simulink model "qless_forgetting_factor_16x16"  (R2021a)
settings: Solver=FixedStepDiscrete  StartTime=0.0  StopTime=stoptime*inf  RelTol=1e-3
InitFcn:
  | qless_init_16chan_fi
undefined symbols (not defined in the file): fc, numArrayElements, physconst, srcAngles, sv, Ts
libraries: hdlsllib x137, commfilt2 x4, commrfcorlib x3, commsync2 x3, commrflib2 x2, commrandsrc3 x2, phasedtxrxlib x2, commdigbbndcpm2 x1, simulink x1, embreciprocals x1, commdigbbndpm3 x1
(part 2 of 22)

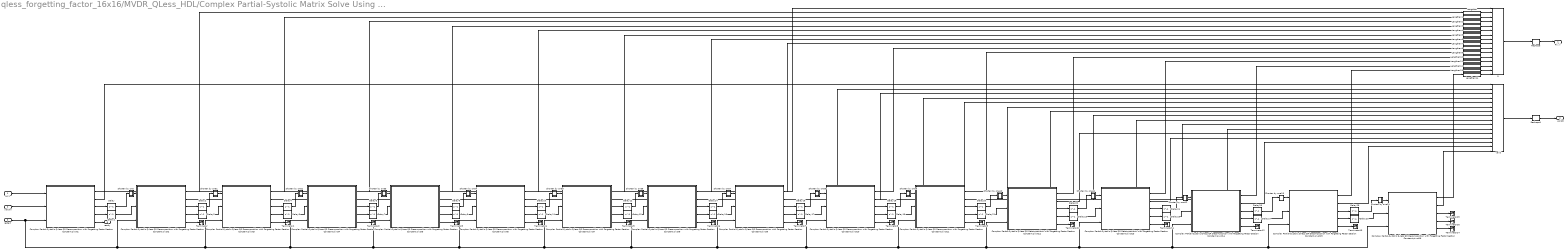
== system qless_forgetting_factor_16x16/MVDR_QLess_HDL/Complex Partial-Systolic Matrix Solve Using Q-less QR Decomposition with Forgetting Factor Manually Tiled n=16/Complex Partial-Systolic Q-less QR with Forgetting Factor/Complex Partial-Systolic Q-less QR with Forgetting Factor Manually tiled ==
  A(i,:) : Inport  PortDimensions=[1,n]
  validIn : Inport  Port=2  PortDimensions=1
  restart : Inport  Port=3  PortDimensions=1
  Complex Partial-Systolic Q-less QR Decomposition with Forgetting Factor Section Constant pivot1 : Subsystem  mask{n=n, forgettingFactor=forgettingFactor, pivot=1}
      mask prompts: n "fixed:emblib:ColumnsInA"; forgettingFactor "fixed:emblib:ForgettingFactor"
      mask DialogControl n Prompt: Number of columns in matrix A
      mask DialogControl forgettingFactor Prompt: Forgetting factor
  Complex Partial-Systolic Q-less QR Decomposition with Forgetting Factor Section Constant pivot10 : Subsystem  mask{n=n-9, forgettingFactor=forgettingFactor, pivot=1}
      mask prompts: n "fixed:emblib:ColumnsInA"; forgettingFactor "fixed:emblib:ForgettingFactor"
      mask DialogControl n Prompt: Number of columns in matrix A
      mask DialogControl forgettingFactor Prompt: Forgetting factor
  Complex Partial-Systolic Q-less QR Decomposition with Forgetting Factor Section Constant pivot11 : Subsystem  mask{n=n-10, forgettingFactor=forgettingFactor, pivot=1}
      mask prompts: n "fixed:emblib:ColumnsInA"; forgettingFactor "fixed:emblib:ForgettingFactor"
      mask DialogControl n Prompt: Number of columns in matrix A
      mask DialogControl forgettingFactor Prompt: Forgetting factor
  Complex Partial-Systolic Q-less QR Decomposition with Forgetting Factor Section Constant pivot12 : Subsystem  mask{n=n-11, forgettingFactor=forgettingFactor, pivot=1}
      mask prompts: n "fixed:emblib:ColumnsInA"; forgettingFactor "fixed:emblib:ForgettingFactor"
      mask DialogControl n Prompt: Number of columns in matrix A
      mask DialogControl forgettingFactor Prompt: Forgetting factor
  Complex Partial-Systolic Q-less QR Decomposition with Forgetting Factor Section Constant pivot13 : Subsystem  mask{n=n-12, forgettingFactor=forgettingFactor, pivot=1}
      mask prompts: n "fixed:emblib:ColumnsInA"; forgettingFactor "fixed:emblib:ForgettingFactor"
      mask DialogControl n Prompt: Number of columns in matrix A
      mask DialogControl forgettingFactor Prompt: Forgetting factor
  Complex Partial-Systolic Q-less QR Decomposition with Forgetting Factor Section Constant pivot14 : Subsystem  mask{n=n-13, forgettingFactor=forgettingFactor, pivot=1}
      mask prompts: n "fixed:emblib:ColumnsInA"; forgettingFactor "fixed:emblib:ForgettingFactor"
      mask DialogControl n Prompt: Number of columns in matrix A
      mask DialogControl forgettingFactor Prompt: Forgetting factor
  Complex Partial-Systolic Q-less QR Decomposition with Forgetting Factor Section Constant pivot15 : Subsystem  mask{n=n-14, forgettingFactor=forgettingFactor, pivot=1}
      mask prompts: n "fixed:emblib:ColumnsInA"; forgettingFactor "fixed:emblib:ForgettingFactor"
      mask DialogControl n Prompt: Number of columns in matrix A
      mask DialogControl forgettingFactor Prompt: Forgetting factor
  Complex Partial-Systolic Q-less QR Decomposition with Forgetting Factor Section Constant pivot16 : Subsystem  mask{n=n-15, forgettingFactor=forgettingFactor, pivot=1}
      mask prompts: n "fixed:emblib:ColumnsInA"; forgettingFactor "fixed:emblib:ForgettingFactor"
      mask DialogControl n Prompt: Number of columns in matrix A
      mask DialogControl forgettingFactor Prompt: Forgetting factor
  Complex Partial-Systolic Q-less QR Decomposition with Forgetting Factor Section Constant pivot2 : Subsystem  mask{n=n-1, forgettingFactor=forgettingFactor, pivot=1}
      mask prompts: n "fixed:emblib:ColumnsInA"; forgettingFactor "fixed:emblib:ForgettingFactor"
      mask DialogControl n Prompt: Number of columns in matrix A
      mask DialogControl forgettingFactor Prompt: Forgetting factor
  Complex Partial-Systolic Q-less QR Decomposition with Forgetting Factor Section Constant pivot3 : Subsystem  mask{n=n-2, forgettingFactor=forgettingFactor, pivot=1}
      mask prompts: n "fixed:emblib:ColumnsInA"; forgettingFactor "fixed:emblib:ForgettingFactor"
      mask DialogControl n Prompt: Number of columns in matrix A
      mask DialogControl forgettingFactor Prompt: Forgetting factor
  Complex Partial-Systolic Q-less QR Decomposition with Forgetting Factor Section Constant pivot4 : Subsystem  mask{n=n-3, forgettingFactor=forgettingFactor, pivot=1}
      mask prompts: n "fixed:emblib:ColumnsInA"; forgettingFactor "fixed:emblib:ForgettingFactor"
      mask DialogControl n Prompt: Number of columns in matrix A
      mask DialogControl forgettingFactor Prompt: Forgetting factor
  Complex Partial-Systolic Q-less QR Decomposition with Forgetting Factor Section Constant pivot5 : Subsystem  mask{n=n-4, forgettingFactor=forgettingFactor, pivot=1}
      mask prompts: n "fixed:emblib:ColumnsInA"; forgettingFactor "fixed:emblib:ForgettingFactor"
      mask DialogControl n Prompt: Number of columns in matrix A
      mask DialogControl forgettingFactor Prompt: Forgetting factor
  Complex Partial-Systolic Q-less QR Decomposition with Forgetting Factor Section Constant pivot6 : Subsystem  mask{n=n-5, forgettingFactor=forgettingFactor, pivot=1}
      mask prompts: n "fixed:emblib:ColumnsInA"; forgettingFactor "fixed:emblib:ForgettingFactor"
      mask DialogControl n Prompt: Number of columns in matrix A
      mask DialogControl forgettingFactor Prompt: Forgetting factor
  Complex Partial-Systolic Q-less QR Decomposition with Forgetting Factor Section Constant pivot7 : Subsystem  mask{n=n-6, forgettingFactor=forgettingFactor, pivot=1}
      mask prompts: n "fixed:emblib:ColumnsInA"; forgettingFactor "fixed:emblib:ForgettingFactor"
      mask DialogControl n Prompt: Number of columns in matrix A
      mask DialogControl forgettingFactor Prompt: Forgetting factor
  Complex Partial-Systolic Q-less QR Decomposition with Forgetting Factor Section Constant pivot8 : Subsystem  mask{n=n-7, forgettingFactor=forgettingFactor, pivot=1}
      mask prompts: n "fixed:emblib:ColumnsInA"; forgettingFactor "fixed:emblib:ForgettingFactor"
      mask DialogControl n Prompt: Number of columns in matrix A
      mask DialogControl forgettingFactor Prompt: Forgetting factor
  Complex Partial-Systolic Q-less QR Decomposition with Forgetting Factor Section Constant pivot9 : Subsystem  mask{n=n-8, forgettingFactor=forgettingFactor, pivot=1}
      mask prompts: n "fixed:emblib:ColumnsInA"; forgettingFactor "fixed:emblib:ForgettingFactor"
      mask DialogControl n Prompt: Number of columns in matrix A
      mask DialogControl forgettingFactor Prompt: Forgetting factor
  Delay{,1..29} (30 alike) : Delay  DelayLength=1
  Lengthen : Subsystem  mask{number_of_leading_zeros=1}
      mask prompts: number_of_leading_zeros "Number of leading zeros to add"
      mask Display: disp('Lengthen')
  Lengthen1 : Subsystem  mask{number_of_leading_zeros=2}
      mask prompts: number_of_leading_zeros "Number of leading zeros to add"
      mask Display: disp('Lengthen')
  Lengthen10 : Subsystem  mask{number_of_leading_zeros=11}
      mask prompts: number_of_leading_zeros "Number of leading zeros to add"
      mask Display: disp('Lengthen')
  Lengthen11 : Subsystem  mask{number_of_leading_zeros=12}
      mask prompts: number_of_leading_zeros "Number of leading zeros to add"
      mask Display: disp('Lengthen')
  Lengthen12 : Subsystem  mask{number_of_leading_zeros=13}
      mask prompts: number_of_leading_zeros "Number of leading zeros to add"
      mask Display: disp('Lengthen')
  Lengthen13 : Subsystem  mask{number_of_leading_zeros=14}
      mask prompts: number_of_leading_zeros "Number of leading zeros to add"
      mask Display: disp('Lengthen')
  Lengthen14 : Subsystem  mask{number_of_leading_zeros=15}
      mask prompts: number_of_leading_zeros "Number of leading zeros to add"
      mask Display: disp('Lengthen')
  Lengthen2 : Subsystem  mask{number_of_leading_zeros=3}
      mask prompts: number_of_leading_zeros "Number of leading zeros to add"
      mask Display: disp('Lengthen')
  Lengthen3 : Subsystem  mask{number_of_leading_zeros=4}
      mask prompts: number_of_leading_zeros "Number of leading zeros to add"
      mask Display: disp('Lengthen')
  Lengthen4 : Subsystem  mask{number_of_leading_zeros=5}
      mask prompts: number_of_leading_zeros "Number of leading zeros to add"
      mask Display: disp('Lengthen')
  Lengthen5 : Subsystem  mask{number_of_leading_zeros=6}
      mask prompts: number_of_leading_zeros "Number of leading zeros to add"
      mask Display: disp('Lengthen')
  Lengthen6 : Subsystem  mask{number_of_leading_zeros=7}
      mask prompts: number_of_leading_zeros "Number of leading zeros to add"
      mask Display: disp('Lengthen')
  Lengthen7 : Subsystem  mask{number_of_leading_zeros=8}
      mask prompts: number_of_leading_zeros "Number of leading zeros to add"
      mask Display: disp('Lengthen')
  Lengthen8 : Subsystem  mask{number_of_leading_zeros=9}
      mask prompts: number_of_leading_zeros "Number of leading zeros to add"
      mask Display: disp('Lengthen')
  Lengthen9 : Subsystem  mask{number_of_leading_zeros=10}
      mask prompts: number_of_leading_zeros "Number of leading zeros to add"
      mask Display: disp('Lengthen')
  R : Concatenate  NumInputs=16
  Reshape : Reshape  OutputDimensionality=Row vector (2-D)
  Reshape1 : Reshape  OutputDimensionality=Row vector (2-D)
  Shorten by one : MATLAB Function  TreatAsAtomicUnit=on
  Shorten by one1 : MATLAB Function  TreatAsAtomicUnit=on
  Shorten by one10 : MATLAB Function  TreatAsAtomicUnit=on
  Shorten by one11 : MATLAB Function  TreatAsAtomicUnit=on
  Shorten by one12 : MATLAB Function  TreatAsAtomicUnit=on
  Shorten by one13 : MATLAB Function  TreatAsAtomicUnit=on
  Shorten by one14 : MATLAB Function  TreatAsAtomicUnit=on
  Shorten by one2 : MATLAB Function  TreatAsAtomicUnit=on
  Shorten by one3 : MATLAB Function  TreatAsAtomicUnit=on
  Shorten by one4 : MATLAB Function  TreatAsAtomicUnit=on
  Shorten by one5 : MATLAB Function  TreatAsAtomicUnit=on
  Shorten by one6 : MATLAB Function  TreatAsAtomicUnit=on
  Shorten by one7 : MATLAB Function  TreatAsAtomicUnit=on
  Shorten by one8 : MATLAB Function  TreatAsAtomicUnit=on
  Shorten by one9 : MATLAB Function  TreatAsAtomicUnit=on
  Terminator{,1..16} (17 alike) : Terminator
  valid : Concatenate  NumInputs=16
  R(i,:).' : Outport  PortDimensions=[1,n*n]
  validR : Outport  Port=2  PortDimensions=[1,n]
  ready : Outport  Port=3  PortDimensions=1
  wires:
  Complex Partial-Systolic Q-less QR Decomposition with Forgetting Factor Section Constant pivot16/1("R(i, :)^T") -> Lengthen14/1(u)
  Lengthen14/1(y) -> R/16
  Shorten by one14/1(y) -> Complex Partial-Systolic Q-less QR Decomposition with Forgetting Factor Section Constant pivot16/1("A(i, :)^T")
  Delay28/1 -> Shorten by one14/1(u)
  Shorten by one13/1(y) -> Complex Partial-Systolic Q-less QR Decomposition with Forgetting Factor Section Constant pivot15/1("A(i, :)^T")
  Delay26/1 -> Shorten by one13/1(u)
  Shorten by one12/1(y) -> Complex Partial-Systolic Q-less QR Decomposition with Forgetting Factor Section Constant pivot14/1("A(i, :)^T")
  Delay24/1 -> Shorten by one12/1(u)
  Shorten by one11/1(y) -> Complex Partial-Systolic Q-less QR Decomposition with Forgetting Factor Section Constant pivot13/1("A(i, :)^T")
  Delay22/1 -> Shorten by one11/1(u)
  Shorten by one10/1(y) -> Complex Partial-Systolic Q-less QR Decomposition with Forgetting Factor Section Constant pivot12/1("A(i, :)^T")
  Delay20/1 -> Shorten by one10/1(u)
  Shorten by one9/1(y) -> Complex Partial-Systolic Q-less QR Decomposition with Forgetting Factor Section Constant pivot11/1("A(i, :)^T")
  Delay18/1 -> Shorten by one9/1(u)
  Shorten by one8/1(y) -> Complex Partial-Systolic Q-less QR Decomposition with Forgetting Factor Section Constant pivot10/1("A(i, :)^T")
  Delay16/1 -> Shorten by one8/1(u)
  Shorten by one7/1(y) -> Complex Partial-Systolic Q-less QR Decomposition with Forgetting Factor Section Constant pivot9/1("A(i, :)^T")
  Delay14/1 -> Shorten by one7/1(u)
  Shorten by one6/1(y) -> Complex Partial-Systolic Q-less QR Decomposition with Forgetting Factor Section Constant pivot8/1("A(i, :)^T")
  Delay12/1 -> Shorten by one6/1(u)
  Shorten by one5/1(y) -> Complex Partial-Systolic Q-less QR Decomposition with Forgetting Factor Section Constant pivot7/1("A(i, :)^T")
  Delay10/1 -> Shorten by one5/1(u)
  Shorten by one4/1(y) -> Complex Partial-Systolic Q-less QR Decomposition with Forgetting Factor Section Constant pivot6/1("A(i, :)^T")
  Delay8/1 -> Shorten by one4/1(u)
  Shorten by one3/1(y) -> Complex Partial-Systolic Q-less QR Decomposition with Forgetting Factor Section Constant pivot5/1("A(i, :)^T")
  Delay6/1 -> Shorten by one3/1(u)
  Delay4/1 -> Shorten by one2/1(u)
  Shorten by one2/1(y) -> Complex Partial-Systolic Q-less QR Decomposition with Forgetting Factor Section Constant pivot4/1("A(i, :)^T")
  Delay2/1 -> Shorten by one1/1(u)
  Shorten by one1/1(y) -> Complex Partial-Systolic Q-less QR Decomposition with Forgetting Factor Section Constant pivot3/1("A(i, :)^T")
  Shorten by one/1(y) -> Complex Partial-Systolic Q-less QR Decomposition with Forgetting Factor Section Constant pivot2/1("A(i, :)^T")
  Lengthen13/1(y) -> R/15
  Lengthen12/1(y) -> R/14
  Lengthen11/1(y) -> R/13
  Lengthen10/1(y) -> R/12
  Lengthen9/1(y) -> R/11
  Lengthen8/1(y) -> R/10
  Lengthen7/1(y) -> R/9
  Lengthen6/1(y) -> R/8
  Lengthen5/1(y) -> R/7
  Lengthen4/1(y) -> R/6
  Lengthen3/1(y) -> R/5
  Lengthen2/1(y) -> R/4
  Lengthen1/1(y) -> R/3
  Lengthen/1(y) -> R/2
  Reshape1/1 -> validR/1
  restart/1 -> Complex Partial-Systolic Q-less QR Decomposition with Forgetting Factor Section Constant pivot1/3(restart), Complex Partial-Systolic Q-less QR Decomposition with Forgetting Factor Section Constant pivot16/3(restart), Complex Partial-Systolic Q-less QR Decomposition with Forgetting Factor Section Constant pivot15/3(restart), Complex Partial-Systolic Q-less QR Decomposition with Forgetting Factor Section Constant pivot14/3(restart), Complex Partial-Systolic Q-less QR Decomposition with Forgetting Factor Section Constant pivot13/3(restart), Complex Partial-Systolic Q-less QR Decomposition with Forgetting Factor Section Constant pivot12/3(restart), Complex Partial-Systolic Q-less QR Decomposition with Forgetting Factor Section Constant pivot11/3(restart), Complex Partial-Systolic Q-less QR Decomposition with Forgetting Factor Section Constant pivot10/3(restart), Complex Partial-Systolic Q-less QR Decomposition with Forgetting Factor Section Constant pivot9/3(restart), Complex Partial-Systolic Q-less QR Decomposition with Forgetting Factor Section Constant pivot8/3(restart), Complex Partial-Systolic Q-less QR Decomposition with Forgetting Factor Section Constant pivot7/3(restart), Complex Partial-Systolic Q-less QR Decomposition with Forgetting Factor Section Constant pivot6/3(restart), Complex Partial-Systolic Q-less QR Decomposition with Forgetting Factor Section Constant pivot5/3(restart), Complex Partial-Systolic Q-less QR Decomposition with Forgetting Factor Section Constant pivot4/3(restart), Complex Partial-Systolic Q-less QR Decomposition with Forgetting Factor Section Constant pivot3/3(restart), Complex Partial-Systolic Q-less QR Decomposition with Forgetting Factor Section Constant pivot2/3(restart)
  valid/1 -> Reshape1/1
  Reshape/1 -> R(i,:).'/1
  R/1 -> Reshape/1
  Complex Partial-Systolic Q-less QR Decomposition with Forgetting Factor Section Constant pivot16/2(validR) -> valid/16
  Complex Partial-Systolic Q-less QR Decomposition with Forgetting Factor Section Constant pivot15/2(validR) -> valid/15
  Complex Partial-Systolic Q-less QR Decomposition with Forgetting Factor Section Constant pivot15/1("R(i, :)^T") -> Lengthen13/1(u)
  Complex Partial-Systolic Q-less QR Decomposition with Forgetting Factor Section Constant pivot14/2(validR) -> valid/14
  Complex Partial-Systolic Q-less QR Decomposition with Forgetting Factor Section Constant pivot14/1("R(i, :)^T") -> Lengthen12/1(u)
  Complex Partial-Systolic Q-less QR Decomposition with Forgetting Factor Section Constant pivot13/2(validR) -> valid/13
  Complex Partial-Systolic Q-less QR Decomposition with Forgetting Factor Section Constant pivot13/1("R(i, :)^T") -> Lengthen11/1(u)
  Complex Partial-Systolic Q-less QR Decomposition with Forgetting Factor Section Constant pivot12/2(validR) -> valid/12
  Complex Partial-Systolic Q-less QR Decomposition with Forgetting Factor Section Constant pivot12/1("R(i, :)^T") -> Lengthen10/1(u)
  Delay29/1 -> Complex Partial-Systolic Q-less QR Decomposition with Forgetting Factor Section Constant pivot16/2(validIn)
  Delay27/1 -> Complex Partial-Systolic Q-less QR Decomposition with Forgetting Factor Section Constant pivot15/2(validIn)
  Delay25/1 -> Complex Partial-Systolic Q-less QR Decomposition with Forgetting Factor Section Constant pivot14/2(validIn)
  Delay23/1 -> Complex Partial-Systolic Q-less QR Decomposition with Forgetting Factor Section Constant pivot13/2(validIn)
  Complex Partial-Systolic Q-less QR Decomposition with Forgetting Factor Section Constant pivot11/2(validR) -> valid/11
  Complex Partial-Systolic Q-less QR Decomposition with Forgetting Factor Section Constant pivot11/1("R(i, :)^T") -> Lengthen9/1(u)
  Complex Partial-Systolic Q-less QR Decomposition with Forgetting Factor Section Constant pivot10/2(validR) -> valid/10
  Complex Partial-Systolic Q-less QR Decomposition with Forgetting Factor Section Constant pivot10/1("R(i, :)^T") -> Lengthen8/1(u)
  Complex Partial-Systolic Q-less QR Decomposition with Forgetting Factor Section Constant pivot9/2(validR) -> valid/9
  Complex Partial-Systolic Q-less QR Decomposition with Forgetting Factor Section Constant pivot9/1("R(i, :)^T") -> Lengthen7/1(u)
  Complex Partial-Systolic Q-less QR Decomposition with Forgetting Factor Section Constant pivot8/2(validR) -> valid/8
  Complex Partial-Systolic Q-less QR Decomposition with Forgetting Factor Section Constant pivot8/1("R(i, :)^T") -> Lengthen6/1(u)
  Complex Partial-Systolic Q-less QR Decomposition with Forgetting Factor Section Constant pivot7/2(validR) -> valid/7
  Complex Partial-Systolic Q-less QR Decomposition with Forgetting Factor Section Constant pivot7/1("R(i, :)^T") -> Lengthen5/1(u)
  Delay21/1 -> Complex Partial-Systolic Q-less QR Decomposition with Forgetting Factor Section Constant pivot12/2(validIn)
  Delay19/1 -> Complex Partial-Systolic Q-less QR Decomposition with Forgetting Factor Section Constant pivot11/2(validIn)
  Delay17/1 -> Complex Partial-Systolic Q-less QR Decomposition with Forgetting Factor Section Constant pivot10/2(validIn)
  Delay15/1 -> Complex Partial-Systolic Q-less QR Decomposition with Forgetting Factor Section Constant pivot9/2(validIn)
  Complex Partial-Systolic Q-less QR Decomposition with Forgetting Factor Section Constant pivot6/2(validR) -> valid/6
  Complex Partial-Systolic Q-less QR Decomposition with Forgetting Factor Section Constant pivot6/1("R(i, :)^T") -> Lengthen4/1(u)
  Delay13/1 -> Complex Partial-Systolic Q-less QR Decomposition with Forgetting Factor Section Constant pivot8/2(validIn)
  Delay11/1 -> Complex Partial-Systolic Q-less QR Decomposition with Forgetting Factor Section Constant pivot7/2(validIn)
  Delay9/1 -> Complex Partial-Systolic Q-less QR Decomposition with Forgetting Factor Section Constant pivot6/2(validIn)
  Complex Partial-Systolic Q-less QR Decomposition with Forgetting Factor Section Constant pivot5/2(validR) -> valid/5
  Complex Partial-Systolic Q-less QR Decomposition with Forgetting Factor Section Constant pivot5/1("R(i, :)^T") -> Lengthen3/1(u)
  Complex Partial-Systolic Q-less QR Decomposition with Forgetting Factor Section Constant pivot4/2(validR) -> valid/4
  Complex Partial-Systolic Q-less QR Decomposition with Forgetting Factor Section Constant pivot4/1("R(i, :)^T") -> Lengthen2/1(u)
  Complex Partial-Systolic Q-less QR Decomposition with Forgetting Factor Section Constant pivot3/2(validR) -> valid/3
  Complex Partial-Systolic Q-less QR Decomposition with Forgetting Factor Section Constant pivot3/1("R(i, :)^T") -> Lengthen1/1(u)
  Delay7/1 -> Complex Partial-Systolic Q-less QR Decomposition with Forgetting Factor Section Constant pivot5/2(validIn)
  Delay5/1 -> Complex Partial-Systolic Q-less QR Decomposition with Forgetting Factor Section Constant pivot4/2(validIn)
  Delay3/1 -> Complex Partial-Systolic Q-less QR Decomposition with Forgetting Factor Section Constant pivot3/2(validIn)
  Complex Partial-Systolic Q-less QR Decomposition with Forgetting Factor Section Constant pivot2/2(validR) -> valid/2
  Complex Partial-Systolic Q-less QR Decomposition with Forgetting Factor Section Constant pivot2/1("R(i, :)^T") -> Lengthen/1(u)
  Delay1/1 -> Complex Partial-Systolic Q-less QR Decomposition with Forgetting Factor Section Constant pivot2/2(validIn)
  Delay/1 -> Shorten by one/1(u)
  Complex Partial-Systolic Q-less QR Decomposition with Forgetting Factor Section Constant pivot1/2(validR) -> valid/1
  Complex Partial-Systolic Q-less QR Decomposition with Forgetting Factor Section Constant pivot1/1("R(i, :)^T") -> R/1
  Complex Partial-Systolic Q-less QR Decomposition with Forgetting Factor Section Constant pivot16/5(ready) -> Terminator14/1
  Complex Partial-Systolic Q-less QR Decomposition with Forgetting Factor Section Constant pivot15/5(ready) -> Terminator13/1
  Complex Partial-Systolic Q-less QR Decomposition with Forgetting Factor Section Constant pivot14/5(ready) -> Terminator12/1
  Complex Partial-Systolic Q-less QR Decomposition with Forgetting Factor Section Constant pivot13/5(ready) -> Terminator11/1
  Complex Partial-Systolic Q-less QR Decomposition with Forgetting Factor Section Constant pivot12/5(ready) -> Terminator10/1
  Complex Partial-Systolic Q-less QR Decomposition with Forgetting Factor Section Constant pivot11/5(ready) -> Terminator9/1
  Complex Partial-Systolic Q-less QR Decomposition with Forgetting Factor Section Constant pivot10/5(ready) -> Terminator8/1
  Complex Partial-Systolic Q-less QR Decomposition with Forgetting Factor Section Constant pivot9/5(ready) -> Terminator7/1
  Complex Partial-Systolic Q-less QR Decomposition with Forgetting Factor Section Constant pivot8/5(ready) -> Terminator6/1
  Complex Partial-Systolic Q-less QR Decomposition with Forgetting Factor Section Constant pivot7/5(ready) -> Terminator5/1
  Complex Partial-Systolic Q-less QR Decomposition with Forgetting Factor Section Constant pivot6/5(ready) -> Terminator4/1
  Complex Partial-Systolic Q-less QR Decomposition with Forgetting Factor Section Constant pivot5/5(ready) -> Terminator3/1
  Complex Partial-Systolic Q-less QR Decomposition with Forgetting Factor Section Constant pivot4/5(ready) -> Terminator2/1
  Complex Partial-Systolic Q-less QR Decomposition with Forgetting Factor Section Constant pivot3/5(ready) -> Terminator1/1
  Complex Partial-Systolic Q-less QR Decomposition with Forgetting Factor Section Constant pivot2/5(ready) -> Terminator/1
  Complex Partial-Systolic Q-less QR Decomposition with Forgetting Factor Section Constant pivot16/4(validY) -> Terminator16/1
  Complex Partial-Systolic Q-less QR Decomposition with Forgetting Factor Section Constant pivot16/3(yOut) -> Terminator15/1
  Complex Partial-Systolic Q-less QR Decomposition with Forgetting Factor Section Constant pivot15/4(validY) -> Delay29/1
  Complex Partial-Systolic Q-less QR Decomposition with Forgetting Factor Section Constant pivot15/3(yOut) -> Delay28/1
  Complex Partial-Systolic Q-less QR Decomposition with Forgetting Factor Section Constant pivot14/3(yOut) -> Delay26/1
  Complex Partial-Systolic Q-less QR Decomposition with Forgetting Factor Section Constant pivot14/4(validY) -> Delay27/1
  Complex Partial-Systolic Q-less QR Decomposition with Forgetting Factor Section Constant pivot13/3(yOut) -> Delay24/1
  Complex Partial-Systolic Q-less QR Decomposition with Forgetting Factor Section Constant pivot13/4(validY) -> Delay25/1
  Complex Partial-Systolic Q-less QR Decomposition with Forgetting Factor Section Constant pivot12/3(yOut) -> Delay22/1
  Complex Partial-Systolic Q-less QR Decomposition with Forgetting Factor Section Constant pivot12/4(validY) -> Delay23/1
  Complex Partial-Systolic Q-less QR Decomposition with Forgetting Factor Section Constant pivot11/3(yOut) -> Delay20/1
  Complex Partial-Systolic Q-less QR Decomposition with Forgetting Factor Section Constant pivot11/4(validY) -> Delay21/1
  Complex Partial-Systolic Q-less QR Decomposition with Forgetting Factor Section Constant pivot10/3(yOut) -> Delay18/1
  Complex Partial-Systolic Q-less QR Decomposition with Forgetting Factor Section Constant pivot10/4(validY) -> Delay19/1
  Complex Partial-Systolic Q-less QR Decomposition with Forgetting Factor Section Constant pivot9/4(validY) -> Delay17/1
  Complex Partial-Systolic Q-less QR Decomposition with Forgetting Factor Section Constant pivot9/3(yOut) -> Delay16/1
  Complex Partial-Systolic Q-less QR Decomposition with Forgetting Factor Section Constant pivot8/4(validY) -> Delay15/1
  Complex Partial-Systolic Q-less QR Decomposition with Forgetting Factor Section Constant pivot8/3(yOut) -> Delay14/1
  Complex Partial-Systolic Q-less QR Decomposition with Forgetting Factor Section Constant pivot7/3(yOut) -> Delay12/1
  Complex Partial-Systolic Q-less QR Decomposition with Forgetting Factor Section Constant pivot7/4(validY) -> Delay13/1
  Complex Partial-Systolic Q-less QR Decomposition with Forgetting Factor Section Constant pivot6/3(yOut) -> Delay10/1
  Complex Partial-Systolic Q-less QR Decomposition with Forgetting Factor Section Constant pivot6/4(validY) -> Delay11/1
  Complex Partial-Systolic Q-less QR Decomposition with Forgetting Factor Section Constant pivot5/3(yOut) -> Delay8/1
  Complex Partial-Systolic Q-less QR Decomposition with Forgetting Factor Section Constant pivot5/4(validY) -> Delay9/1
  Complex Partial-Systolic Q-less QR Decomposition with Forgetting Factor Section Constant pivot4/3(yOut) -> Delay6/1
  Complex Partial-Systolic Q-less QR Decomposition with Forgetting Factor Section Constant pivot4/4(validY) -> Delay7/1
  Complex Partial-Systolic Q-less QR Decomposition with Forgetting Factor Section Constant pivot3/3(yOut) -> Delay4/1
  Complex Partial-Systolic Q-less QR Decomposition with Forgetting Factor Section Constant pivot3/4(validY) -> Delay5/1
  Complex Partial-Systolic Q-less QR Decomposition with Forgetting Factor Section Constant pivot2/3(yOut) -> Delay2/1
  Complex Partial-Systolic Q-less QR Decomposition with Forgetting Factor Section Constant pivot2/4(validY) -> Delay3/1
  Complex Partial-Systolic Q-less QR Decomposition with Forgetting Factor Section Constant pivot1/4(validY) -> Delay1/1
  Complex Partial-Systolic Q-less QR Decomposition with Forgetting Factor Section Constant pivot1/3(yOut) -> Delay/1
  Complex Partial-Systolic Q-less QR Decomposition with Forgetting Factor Section Constant pivot1/5(ready) -> ready/1
  validIn/1 -> Complex Partial-Systolic Q-less QR Decomposition with Forgetting Factor Section Constant pivot1/2(validIn)
  A(i,:)/1 -> Complex Partial-Systolic Q-less QR Decomposition with Forgetting Factor Section Constant pivot1/1("A(i, :)^T")

== system qless_forgetting_factor_16x16/MVDR_QLess_HDL/Complex Partial-Systolic Matrix Solve Using Q-less QR Decomposition with Forgetting Factor Manually Tiled n=16/Complex Partial-Systolic Q-less QR with Forgetting Factor/Partial-Systolic Q-less QR with Forgetting Factor Output Memory Manager ==
  RtransposeIn : Inport
  validIn : Inport  Port=2
  restart : Inport  Port=3
  Partial-Systolic Q-less QR Output Memory Manager1 : Subsystem  mask{m=n, n=n}
      mask prompts: m "fixed:emblib:RowsInA"; n "fixed:emblib:ColumnsInA"
      mask DialogControl m Prompt: Number of rows in matrix A
      mask DialogControl n Prompt: Number of columns in matrix A
      mask Display: disp('QR Output Memory Manager')
  RtransposeOut : Outport
  validOut : Outport  Port=2
  wires:
  validIn/1 -> Partial-Systolic Q-less QR Output Memory Manager1/2(validIn)
  Partial-Systolic Q-less QR Output Memory Manager1/2(validOut) -> validOut/1
  Partial-Systolic Q-less QR Output Memory Manager1/1(RtransposeOut) -> RtransposeOut/1
  RtransposeIn/1 -> Partial-Systolic Q-less QR Output Memory Manager1/1(RtransposeIn)
  restart/1 -> Partial-Systolic Q-less QR Output Memory Manager1/3(restart)

== system qless_forgetting_factor_16x16/MVDR_QLess_HDL/Complex Partial-Systolic Matrix Solve Using Q-less QR Decomposition with Forgetting Factor Manually Tiled n=16/Complex Q-less QR Forward Backward Substitute/Complex Burst Back Substitute with Matrix Output1 ==
  "R(i, :)" : Inport
  "C(i, :)" : Inport  Port=2
  validIn : Inport  Port=3
  start : Inport  Port=4
  restart : Inport  Port=5
  Back substitute logic : Subsystem  TreatAsAtomicUnit=on
  Cast : DataTypeConversion  OutDataTypeStr=OutputType
  Cast to Union of Types : MATLAB Function  TreatAsAtomicUnit=on
  Cast1 : DataTypeConversion  OutDataTypeStr=int32
  Delay : Delay  DelayLength=1
  Delay One Step{,1..3} (4 alike) : Delay  DelayLength=1
  Reciprocal of the diagonal element : Subsystem
  X : Outport  VectorParamsAs1DForOutWhenUnconnected=off
  validOut : Outport  Port=2  VectorParamsAs1DForOutWhenUnconnected=off
  rowReady : Outport  Port=3  VectorParamsAs1DForOutWhenUnconnected=off
  ready : Outport  Port=4  VectorParamsAs1DForOutWhenUnconnected=off
  wires:
  restart/1 -> Delay/1
  Delay/1 -> Back substitute logic/7(restart)
  Delay One Step3/1 -> Cast to Union of Types/1(Xref)
  "C(i, :)"/1 -> Cast to Union of Types/2(Cin)
  Cast/1 -> X/1, Delay One Step3/1
  start/1 -> Back substitute logic/6(start), Reciprocal of the diagonal element/2(start)
  Reciprocal of the diagonal element/3(validOut) -> Delay One Step2/1
  Reciprocal of the diagonal element/1(inverseElement) -> Delay One Step/1
  Cast to Union of Types/1(Cout) -> Back substitute logic/4(cIn)
  validIn/1 -> Reciprocal of the diagonal element/3(validIn)
  Delay One Step1/1 -> Cast1/1
  Cast1/1 -> Back substitute logic/2(inverseShift)
  Delay One Step/1 -> Back substitute logic/1(inverseElement)
  Reciprocal of the diagonal element/2(inverseShift) -> Delay One Step1/1
  Delay One Step2/1 -> Back substitute logic/5(validIn)
  "R(i, :)"/1 -> Reciprocal of the diagonal element/1(rIn), Back substitute logic/3(rIn)
  Back substitute logic/1(X) -> Cast/1
  Back substitute logic/2(validOut) -> validOut/1
  Back substitute logic/3(rowReady) -> rowReady/1
  Back substitute logic/4(ready) -> ready/1

== system qless_forgetting_factor_16x16/MVDR_QLess_HDL/Complex Partial-Systolic Matrix Solve Using Q-less QR Decomposition with Forgetting Factor Manually Tiled n=16/Complex Q-less QR Forward Backward Substitute/Complex Burst Forward Substitute with Matrix Output ==
  "L(i, :)" : Inport
  "C(i, :)" : Inport  Port=2
  validIn : Inport  Port=3
  start : Inport  Port=4
  restart : Inport  Port=5
  Cast : DataTypeConversion  OutDataTypeStr=OutputType
  Cast to Union of Types : MATLAB Function  TreatAsAtomicUnit=on
  Cast1 : DataTypeConversion  OutDataTypeStr=int32
  Delay : Delay  DelayLength=1
  Delay One Step{,1..3} (4 alike) : Delay  DelayLength=1
  Forward substitute logic : Subsystem  TreatAsAtomicUnit=on
  Reciprocal of the diagonal element : Subsystem
  X : Outport  VectorParamsAs1DForOutWhenUnconnected=off
  validOut : Outport  Port=2  VectorParamsAs1DForOutWhenUnconnected=off
  rowReady : Outport  Port=3  VectorParamsAs1DForOutWhenUnconnected=off
  ready : Outport  Port=4  VectorParamsAs1DForOutWhenUnconnected=off
  wires:
  restart/1 -> Delay/1
  Delay/1 -> Forward substitute logic/7(restart)
  Delay One Step3/1 -> Cast to Union of Types/1(Xref)
  "C(i, :)"/1 -> Cast to Union of Types/2(Cin)
  Cast/1 -> X/1, Delay One Step3/1
  start/1 -> Forward substitute logic/6(start), Reciprocal of the diagonal element/2(start)
  Reciprocal of the diagonal element/3(validOut) -> Delay One Step2/1
  Reciprocal of the diagonal element/1(inverseElement) -> Delay One Step/1
  Cast to Union of Types/1(Cout) -> Forward substitute logic/4(cIn)
  validIn/1 -> Reciprocal of the diagonal element/3(validIn)
  Delay One Step1/1 -> Cast1/1
  Cast1/1 -> Forward substitute logic/2(inverseShift)
  Delay One Step/1 -> Forward substitute logic/1(inverseElement)
  Reciprocal of the diagonal element/2(inverseShift) -> Delay One Step1/1
  Delay One Step2/1 -> Forward substitute logic/5(validIn)
  "L(i, :)"/1 -> Reciprocal of the diagonal element/1(rIn), Forward substitute logic/3(rIn)
  Forward substitute logic/1(X) -> Cast/1
  Forward substitute logic/2(validOut) -> validOut/1
  Forward substitute logic/3(rowReady) -> rowReady/1
  Forward substitute logic/4(ready) -> ready/1

== system qless_forgetting_factor_16x16/MVDR_QLess_HDL/Complex Partial-Systolic Matrix Solve Using Q-less QR Decomposition with Forgetting Factor Manually Tiled n=16/Complex Q-less QR Forward Backward Substitute/Partial-Systolic Matrix Solve Q-less QR B Buffer Manager ==
  rowForFwdSub : Inport
  fwdSubValidIn : Inport  Port=2
  B : Inport  Port=3
  bValidIn : Inport  Port=4
  backSubDone : Inport  Port=5
  restart : Inport  Port=6
  B Buffer Manager State Machine : MATLAB Function  TreatAsAtomicUnit=on  mask{n=n}
      mask prompts: n "fixed:emblib:ColumnsInA"
  Reshape : Reshape  OutputDimensionality=Customize  OutputDimensions=[n,p]
  Reshape2 : Reshape  OutputDimensionality=Column vector (2-D)
  Reshape4 : Reshape  OutputDimensionality=Row vector (2-D)
  Save Matrix B : Subsystem  mask{n=n}
      mask prompts: n "fixed:emblib:ColumnsInA"
      mask help: The n-by-n input matrix is flattened to an1-by-n^2 row. The row selector is a 1-by-n vector of logical values with a true element corresponding to a row of the matrix to save. There is one cycle delay between input and output.
      mask DialogControl n Prompt: Number of columns in matrix A
      mask Display: disp('Save matrix')
  Select row R(i,:) : Selector  NumberOfDimensions=2  InputPortWidth=3  IndexOptions=Starting index (port),Select all  Indices=1:n,1  OutputSizes=1,1
  lRow : Outport
  cRow : Outport  Port=2
  validOut : Outport  Port=3
  start : Outport  Port=4
  readyForFwdSub : Outport  Port=5
  wires:
  B Buffer Manager State Machine/5(readyForFwdSub) -> readyForFwdSub/1
  B Buffer Manager State Machine/4(start) -> start/1
  B Buffer Manager State Machine/3(validOut) -> validOut/1
  Reshape4/1 -> cRow/1
  B Buffer Manager State Machine/1(Lrow) -> lRow/1
  B Buffer Manager State Machine/2(rowIndex) -> Select row R(i,:)/2
  Save Matrix B/1(matrixOut) -> Reshape/1
  Reshape/1 -> Select row R(i,:)/1
  Select row R(i,:)/1 -> Reshape4/1
  Reshape2/1 -> Save Matrix B/1(matrixIn)
  backSubDone/1 -> B Buffer Manager State Machine/4(backSubDone)
  B/1 -> Reshape2/1
  fwdSubValidIn/1 -> B Buffer Manager State Machine/2(fwdSubValidIn)
  restart/1 -> B Buffer Manager State Machine/5(restart), Save Matrix B/3(restart)
  bValidIn/1 -> B Buffer Manager State Machine/3(bValidIn), Save Matrix B/2(validIn)
  rowForFwdSub/1 -> B Buffer Manager State Machine/1(rowForFwdSub)

== system qless_forgetting_factor_16x16/MVDR_QLess_HDL/Complex Partial-Systolic Matrix Solve Using Q-less QR Decomposition with Forgetting Factor Manually Tiled n=16/Complex Q-less QR Forward Backward Substitute/Partial-Systolic Matrix Solve Q-less QR Forward Substitute Memory Manager ==
  inputMatrix : Inport
  inputValidIn : Inport  Port=2
  needFwdSubRow : Inport  Port=3
  backSubDone : Inport  Port=4
  restart : Inport  Port=5
  MATLAB Function1 : MATLAB Function  TreatAsAtomicUnit=on  mask{n=n}
      mask prompts: n "fixed:emblib:ColumnsInA"
  Reshape : Reshape  OutputDimensionality=Customize  OutputDimensions=[n,p]
  Reshape2 : Reshape  OutputDimensionality=Column vector (2-D)
  Reshape4 : Reshape  OutputDimensionality=Row vector (2-D)
  Save Matrix B : Subsystem  mask{n=n}
      mask prompts: n "fixed:emblib:ColumnsInA"
      mask help: The n-by-n input matrix is flattened to an1-by-n^2 row. The row selector is a 1-by-n vector of logical values with a true element corresponding to a row of the matrix to save. There is one cycle delay between input and output.
      mask DialogControl n Prompt: Number of columns in matrix A
      mask Display: disp('Save matrix')
  Select row R(i,:) : Selector  NumberOfDimensions=2  InputPortWidth=3  IndexOptions=Starting index (port),Select all  Indices=1:n,1  OutputSizes=1,1
  fwdSubRow : Outport
  fwdSubValidIn : Outport  Port=2
  needBackSubRow : Outport  Port=3
  wires:
  MATLAB Function1/3(needBackSubRow) -> needBackSubRow/1
  MATLAB Function1/2(validOut) -> fwdSubValidIn/1
  Reshape4/1 -> fwdSubRow/1
  needFwdSubRow/1 -> MATLAB Function1/2(needFwdSubRow)
  MATLAB Function1/1(rowIndex) -> Select row R(i,:)/2
  Save Matrix B/1(matrixOut) -> Reshape/1
  Reshape/1 -> Select row R(i,:)/1
  Select row R(i,:)/1 -> Reshape4/1
  Reshape2/1 -> Save Matrix B/1(matrixIn)
  backSubDone/1 -> MATLAB Function1/3(backSubDone)
  inputMatrix/1 -> Reshape2/1
  restart/1 -> Save Matrix B/3(restart), MATLAB Function1/4(restart)
  inputValidIn/1 -> MATLAB Function1/1(inputValidIn), Save Matrix B/2(validIn)

== system qless_forgetting_factor_16x16/MVDR_QLess_HDL/Complex Partial-Systolic Matrix Solve Using Q-less QR Decomposition with Forgetting Factor Manually Tiled n=16/Complex Q-less QR Forward Backward Substitute/Partial-Systolic Matrix Solve Q-less QR Output Manager ==
  rMatrix : Inport
  validInR : Inport  Port=2
  backSubDone : Inport  Port=3
  restart : Inport  Port=4
  needRowBackSub : Inport  Port=5
  needRowFwdSub : Inport  Port=6
  readyForFwdSub : Inport  Port=7
  Conjugate : Math  Operator=conj  SignedPower=on  RndMeth=Zero  SaturateOnIntegerOverflow=on
  Partial-Systolic Manage QR Output State Machine : MATLAB Function  TreatAsAtomicUnit=on  mask{n=n}
      mask prompts: n "fixed:emblib:ColumnsInA"
  Reshape : Reshape  OutputDimensionality=Customize  OutputDimensions=[n, n]
  Reshape1 : Reshape  OutputDimensionality=Row vector (2-D)
  Reshape2 : Reshape  OutputDimensionality=Column vector (2-D)
  Reshape4 : Reshape  OutputDimensionality=Row vector (2-D)
  Save Matrix : Subsystem  mask{n=n}
      mask prompts: n "fixed:emblib:ColumnsInA"
      mask help: The n-by-n input matrix is flattened to an1-by-n^2 row. The row selector is a 1-by-n vector of logical values with a true element corresponding to a row of the matrix to save. There is one cycle delay between input and output.
      mask DialogControl n Prompt: Number of columns in matrix A
      mask Display: disp('Save matrix')
  Select column : Selector  NumberOfDimensions=2  InputPortWidth=3  IndexOptions=Select all,Starting index (port)  Indices=1:n,1  OutputSizes=1,1
  Select row : Selector  NumberOfDimensions=2  InputPortWidth=3  IndexOptions=Starting index (port),Select all  Indices=1:n,1  OutputSizes=1,1
  columnForFwdSub : Outport
  fwdSubValidOut : Outport  Port=2
  rowForBackSub : Outport  Port=3
  wires:
  Partial-Systolic Manage QR Output State Machine/1(columnOutIndex) -> Select column/2
  Partial-Systolic Manage QR Output State Machine/3(rowOutIndex) -> Select row/2
  Partial-Systolic Manage QR Output State Machine/5(restartOut) -> Save Matrix/3(restart)
  Partial-Systolic Manage QR Output State Machine/4(validR) -> Save Matrix/2(validIn)
  Reshape/1 -> Select column/1, Select row/1
  Reshape4/1 -> rowForBackSub/1
  Reshape1/1 -> columnForFwdSub/1
  Select row/1 -> Reshape4/1
  Reshape2/1 -> Save Matrix/1(matrixIn)
  Save Matrix/1(matrixOut) -> Reshape/1
  Conjugate/1 -> Reshape1/1
  Select column/1 -> Conjugate/1
  validInR/1 -> Partial-Systolic Manage QR Output State Machine/1(validIn)
  restart/1 -> Partial-Systolic Manage QR Output State Machine/5(restartIn)
  rMatrix/1 -> Reshape2/1
  needRowBackSub/1 -> Partial-Systolic Manage QR Output State Machine/3(needRowBackSub)
  needRowFwdSub/1 -> Partial-Systolic Manage QR Output State Machine/2(needRowFwdSub)
  readyForFwdSub/1 -> Partial-Systolic Manage QR Output State Machine/6(readyForFwdSub)
  Partial-Systolic Manage QR Output State Machine/2(fwdSubValidOut) -> fwdSubValidOut/1
  backSubDone/1 -> Partial-Systolic Manage QR Output State Machine/4(backSubDone)

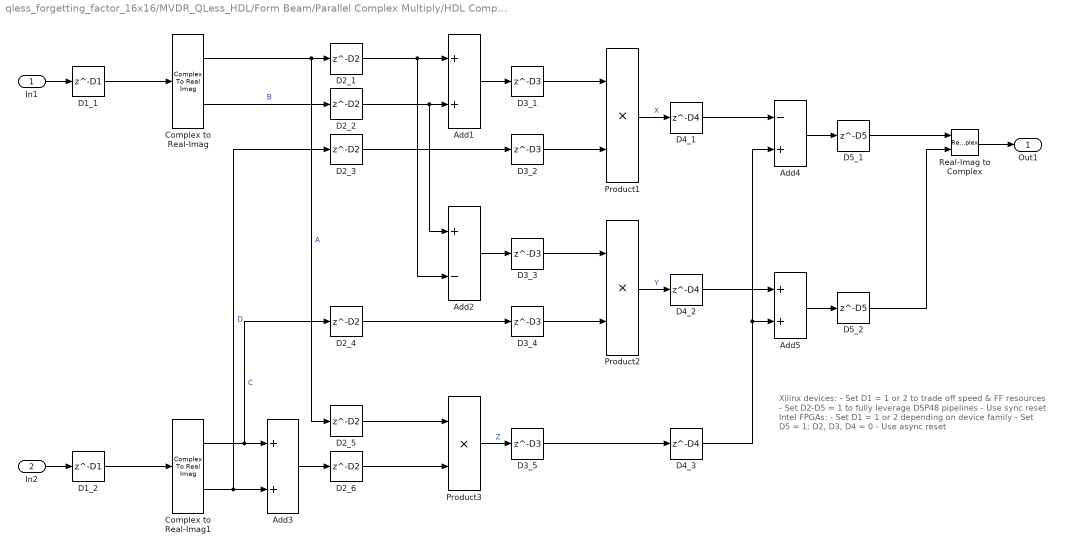
== system qless_forgetting_factor_16x16/MVDR_QLess_HDL/Form Beam/Parallel Complex Multiply/HDL Complex Multiply ==
  note: Xilinx devices:
      | - Set D1 = 1 or 2 to trade off speed & FF resources
      | - Set D2-D5 = 1 to fully leverage DSP48 pipelines
      | - Use sync reset
      |
      | Intel FPGAs:
      | - Set D1 = 1 or 2 depending on device family
      | - Set D5 = 1; D2, D3, D4 = 0
      | - Use async reset
  In1 : Inport
  In2 : Inport  Port=2
  Add1 : Sum
  Add2 : Sum  Inputs=+-
  Add3 : Sum
  Add4 : Sum  Inputs=-+
  Add5 : Sum
  Complex to Real-Imag : ComplexToRealImag
  Complex to Real-Imag1 : ComplexToRealImag
  D1_1 : Delay  DelayLength=D1
  D1_2 : Delay  DelayLength=D1
  D2_{1..6} (6 alike) : Delay  DelayLength=D2
  D3_{1..5} (5 alike) : Delay  DelayLength=D3
  D4_1 : Delay  DelayLength=D4
  D4_2 : Delay  DelayLength=D4
  D4_3 : Delay  DelayLength=D4
  D5_1 : Delay  DelayLength=D5
  D5_2 : Delay  DelayLength=D5
  Product1 : Product
  Product2 : Product
  Product3 : Product
  Real-Imag to Complex : RealImagToComplex
  Out1 : Outport  VectorParamsAs1DForOutWhenUnconnected=off
  wires:
  Real-Imag to Complex/1 -> Out1/1
  In2/1 -> D1_2/1
  Complex to Real-Imag1/1 -> Add3/1, D2_4/1  "C"
  Complex to Real-Imag1/2 -> Add3/2, D2_3/1  "D"
  Product1/1 -> D4_1/1  "X"
  Product2/1 -> D4_2/1  "Y"
  Product3/1 -> D3_5/1  "Z"
  Add4/1 -> D5_1/1
  Add5/1 -> D5_2/1
  D5_1/1 -> Real-Imag to Complex/1
  D5_2/1 -> Real-Imag to Complex/2
  D4_1/1 -> Add4/1
  D4_2/1 -> Add5/1
  D3_5/1 -> D4_3/1
  Add1/1 -> D3_1/1
  Add3/1 -> D2_6/1
  Add2/1 -> D3_3/1
  Complex to Real-Imag/1 -> D2_5/1, D2_1/1  "A"
  Complex to Real-Imag/2 -> D2_2/1  "B"
  D3_1/1 -> Product1/1
  D2_6/1 -> Product3/2
  D3_3/1 -> Product2/1
  D4_3/1 -> Add4/2, Add5/2
  D3_4/1 -> Product2/2
  D3_2/1 -> Product1/2
  D2_4/1 -> D3_4/1
  D2_3/1 -> D3_2/1
  D2_5/1 -> Product3/1
  D2_2/1 -> Add1/2, Add2/1
  D2_1/1 -> Add2/2, Add1/1
  In1/1 -> D1_1/1
  D1_1/1 -> Complex to Real-Imag/1
  D1_2/1 -> Complex to Real-Imag1/1

== system qless_forgetting_factor_16x16/MVDR_QLess_HDL/Normalize Response/MVDR Weight Update/Inner Product ==
  u : Inport
  v : Inport  Port=2
  validIn : Inport  Port=3
  Conjugate : Math  Operator=conj  SignedPower=on  RndMeth=Zero  SaturateOnIntegerOverflow=on
  Delay : Delay  DelayLength=1
  Delay1 : Delay  DelayLength=6
  Delay2 : Delay  DelayLength=ceil(log2(numArrayElements))
  Delay4 : Delay  DelayLength=1
  Element-wise complex product : Subsystem  TreatAsAtomicUnit=on
  Tree Sum with Distributed Pipelining : Subsystem
  y : Outport
  validOut : Outport  Port=2
  wires:
  v/1 -> Conjugate/1
  u/1 -> Element-wise complex product/2(v)
  validIn/1 -> Delay1/1
  Element-wise complex product/1(y) -> Delay/1
  Delay2/1 -> validOut/1
  Delay1/1 -> Delay4/1
  Delay4/1 -> Delay2/1
  Conjugate/1 -> Element-wise complex product/1(u)
  Delay/1 -> Tree Sum with Distributed Pipelining/1(In1)
  Tree Sum with Distributed Pipelining/1(Out1) -> y/1

== system qless_forgetting_factor_16x16/MVDR_QLess_HDL/Normalize Response/MVDR Weight Update/Vector // Scalar Divide ==
  x : Inport
  y : Inport  Port=2
  validIn : Inport  Port=3
  Complex to Real-Imag : ComplexToRealImag  Output=Real
  Data Type Conversion : DataTypeConversion  OutDataTypeStr=fixdt(1,18,16)
  Delay{1..6,11..13} (9 alike) : Delay  DelayLength=1
  Delay{7..10} (4 alike) : Delay
  Delay14 : Delay  DelayLength=34
  MATLAB Function : MATLAB Function  TreatAsAtomicUnit=on
  Normalized Reciprocal HDL Optimized : embreciprocals/Normalized Reciprocal HDL Optimized
      settings: SourceProductBaseCode=SL
  Product : Product  OutDataTypeStr=Inherit: Same as first input
  w : Outport
  validOut : Outport  Port=2
  wires:
  Delay2/1 -> MATLAB Function/2(e)
  y/1 -> Complex to Real-Imag/1
  Delay12/1 -> Data Type Conversion/1
  Complex to Real-Imag/1 -> Normalized Reciprocal HDL Optimized/1
  Delay13/1 -> Delay7/1
  Normalized Reciprocal HDL Optimized/2 -> Delay11/1
  Normalized Reciprocal HDL Optimized/1 -> Delay12/1
  Delay1/1 -> MATLAB Function/1(y)
  validIn/1 -> Normalized Reciprocal HDL Optimized/2
  Product/1 -> Delay1/1
  Delay11/1 -> Delay9/1
  MATLAB Function/1(w) -> Delay3/1
  Normalized Reciprocal HDL Optimized/3 -> Delay4/1
  Delay3/1 -> w/1
  Delay4/1 -> Delay10/1
  Delay5/1 -> Delay6/1
  Delay6/1 -> validOut/1
  x/1 -> Delay14/1
  Data Type Conversion/1 -> Delay8/1
  Delay7/1 -> Product/1
  Delay8/1 -> Product/2
  Delay9/1 -> Delay2/1
  Delay10/1 -> Delay5/1
  Delay14/1 -> Delay13/1

== system qless_forgetting_factor_16x16/MVDR_QLess_HDL/Complex Partial-Systolic Matrix Solve Using Q-less QR Decomposition with Forgetting Factor Manually Tiled n=16/Complex Partial-Systolic Q-less QR with Forgetting Factor/Complex Partial-Systolic Q-less QR with Forgetting Factor Manually tiled/Complex Partial-Systolic Q-less QR Decomposition with Forgetting Factor Section Constant pivot1 ==
  "A(i, :)^T" : Inport
  validIn : Inport  Port=2
  restart : Inport  Port=3
  Complex Partial-Systolic Q-less QR Row Rotations : Subsystem  mask(QR Complex Row Rotations){n=n, pivot=pivot}
      mask prompts: n "fixed:emblib:ColumnsInA"
      mask help: fixed:emblib:ComplexRowRotationsFullDescription
      mask DialogControl n Prompt: Number of columns in matrix A
  Data Type Conversion{,2..6} (6 alike) : DataTypeConversion  OutDataTypeStr=boolean
  Forgetting Factor : Gain  Gain=forgettingFactor  OutDataTypeStr=Inherit: Same as input
  Partial-Systolic Q-less QR with Forgetting Factor Memory Controller : Subsystem  TreatAsAtomicUnit=on  mask(Burst Q-less QR QR Memory Controller){n=n}
      mask prompts: n "fixed:emblib:ColumnsInA"
      mask help: fixed:emblib:MemoryControllerDescription
      mask DialogControl n Prompt: Number of columns in matrix A
  Same Datatype : Subsystem  TreatAsAtomicUnit=on
  Terminator : Terminator
  "R(i, :)^T" : Outport  VectorParamsAs1DForOutWhenUnconnected=off
  validR : Outport  Port=2  VectorParamsAs1DForOutWhenUnconnected=off
  yOut : Outport  Port=3  VectorParamsAs1DForOutWhenUnconnected=off
  validY : Outport  Port=4  VectorParamsAs1DForOutWhenUnconnected=off
  ready : Outport  Port=5  VectorParamsAs1DForOutWhenUnconnected=off
  wires:
  "A(i, :)^T"/1 -> Same Datatype/2(Reference), Partial-Systolic Q-less QR with Forgetting Factor Memory Controller/2(aIn)
  restart/1 -> Data Type Conversion2/1
  Complex Partial-Systolic Q-less QR Row Rotations/3(validOut) -> Data Type Conversion3/1
  Partial-Systolic Q-less QR with Forgetting Factor Memory Controller/4(validOut) -> Data Type Conversion5/1
  validIn/1 -> Data Type Conversion/1
  Partial-Systolic Q-less QR with Forgetting Factor Memory Controller/2(yOut) -> Complex Partial-Systolic Q-less QR Row Rotations/2(y)
  Same Datatype/1(DataOut) -> Partial-Systolic Q-less QR with Forgetting Factor Memory Controller/1(xIn)
  Partial-Systolic Q-less QR with Forgetting Factor Memory Controller/5(ready) -> Data Type Conversion6/1
  Complex Partial-Systolic Q-less QR Row Rotations/2(yOut) -> yOut/1
  Complex Partial-Systolic Q-less QR Row Rotations/4(ready) -> Terminator/1
  Partial-Systolic Q-less QR with Forgetting Factor Memory Controller/3(process) -> Data Type Conversion4/1
  Complex Partial-Systolic Q-less QR Row Rotations/1(xOut) -> Forgetting Factor/1
  Partial-Systolic Q-less QR with Forgetting Factor Memory Controller/1(xOut) -> Complex Partial-Systolic Q-less QR Row Rotations/1(x), "R(i, :)^T"/1
  Forgetting Factor/1 -> Same Datatype/1(Data)
  Data Type Conversion/1 -> Partial-Systolic Q-less QR with Forgetting Factor Memory Controller/3(validIn)
  Data Type Conversion2/1 -> Complex Partial-Systolic Q-less QR Row Rotations/4(restart), Partial-Systolic Q-less QR with Forgetting Factor Memory Controller/5(restart)
  Data Type Conversion3/1 -> Partial-Systolic Q-less QR with Forgetting Factor Memory Controller/4(validElim), validY/1
  Data Type Conversion5/1 -> validR/1
  Data Type Conversion6/1 -> ready/1
  Data Type Conversion4/1 -> Complex Partial-Systolic Q-less QR Row Rotations/3(validIn)
